simulink model "lab4p2b"  (R2023b)
settings: Solver=ode23tb  StartTime=0.0  StopTime=Tmdl  FixedStep=To/100  MaxStep=To/100  RelTol=1e-3
undefined symbols (not defined in the file or in its folder): an, dsc, T, To
settings Model: Creator=deniskirbaba  LastModifiedBy=Max

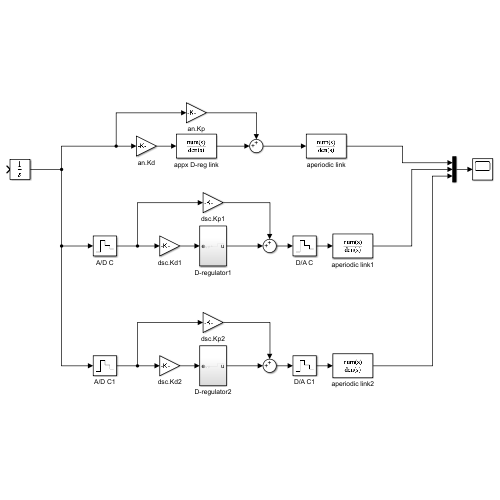
[thumbnail: Simulink's stored preview of the top-level diagram]
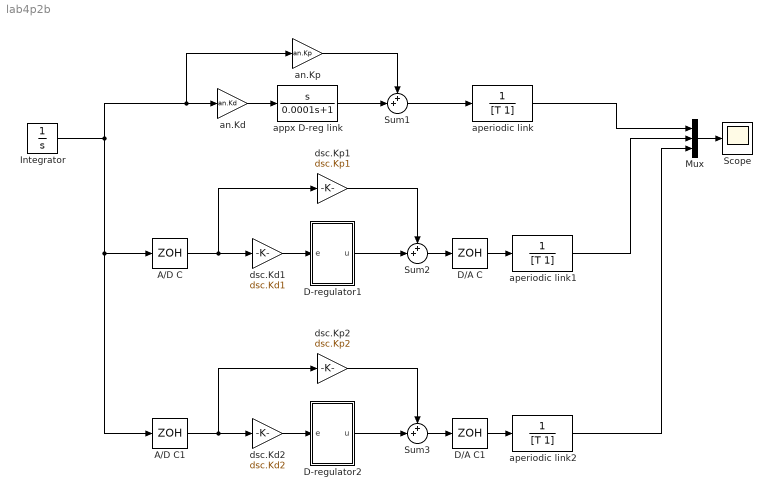
== system lab4p2b ==
  A/D C : ZeroOrderHold  SampleTime=To
  A/D C1 : ZeroOrderHold  SampleTime=To
  D-regulator1 : Subsystem
  D-regulator2 : Subsystem
  D/A C : ZeroOrderHold  SampleTime=To
  D/A C1 : ZeroOrderHold  SampleTime=To
  Integrator : Integrator  InitialCondition=1
  Mux : Mux  Inputs=3
  Scope : Scope
  Sum1 : Sum  Inputs=++|
  Sum2 : Sum  Inputs=++|
  Sum3 : Sum  Inputs=++|
  an.Kd : Gain  Gain=an.Kd
  an.Kp : Gain  Gain=an.Kp
  aperiodic link : TransferFcn  Denominator=[T 1]
  aperiodic link1 : TransferFcn  Denominator=[T 1]
  aperiodic link2 : TransferFcn  Denominator=[T 1]
  appx D-reg link : TransferFcn  Numerator=[1 0]  Denominator=[0.0001 1]
  dsc.Kd1 : Gain  Gain=dsc.Kd1
  dsc.Kd2 : Gain  Gain=dsc.Kd2
  dsc.Kp1 : Gain  Gain=dsc.Kp1
  dsc.Kp2 : Gain  Gain=dsc.Kp2
  wires:
  an.Kd/1 -> appx D-reg link/1
  Mux/1 -> Scope/1
  appx D-reg link/1 -> Sum1/2
  an.Kp/1 -> Sum1/1
  Sum1/1 -> aperiodic link/1
  aperiodic link/1 -> Mux/1
  dsc.Kd1/1 -> D-regulator1/1(e)
  D-regulator1/1(u) -> Sum2/2
  A/D C/1 -> dsc.Kp1/1, dsc.Kd1/1
  dsc.Kp1/1 -> Sum2/1
  Sum2/1 -> D/A C/1
  aperiodic link1/1 -> Mux/2
  D/A C/1 -> aperiodic link1/1
  aperiodic link2/1 -> Mux/3
  D/A C1/1 -> aperiodic link2/1
  dsc.Kp2/1 -> Sum3/1
  A/D C1/1 -> dsc.Kp2/1, dsc.Kd2/1
  Sum3/1 -> D/A C1/1
  dsc.Kd2/1 -> D-regulator2/1(e)
  D-regulator2/1(u) -> Sum3/2
  Integrator/1 -> A/D C1/1, A/D C/1, an.Kp/1, an.Kd/1

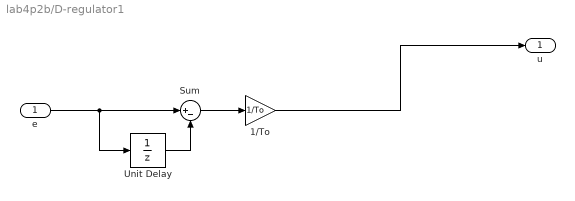
== system lab4p2b/D-regulator1 ==
  e : Inport
  1/To : Gain  Gain=1/To
  Sum : Sum  Inputs=|+-
  Unit Delay : UnitDelay  SampleTime=To  HasFrameUpgradeWarning=on
  u : Outport
  wires:
  1/To/1 -> u/1
  Unit Delay/1 -> Sum/2
  e/1 -> Unit Delay/1, Sum/1
  Sum/1 -> 1/To/1

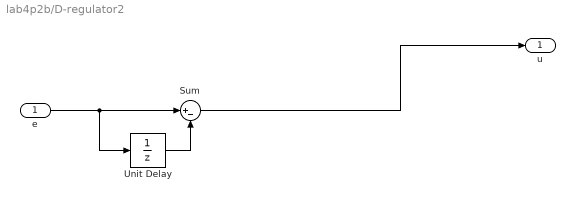
== system lab4p2b/D-regulator2 ==
  e : Inport
  Sum : Sum  Inputs=|+-
  Unit Delay : UnitDelay  SampleTime=To  HasFrameUpgradeWarning=on
  u : Outport
  wires:
  Sum/1 -> u/1
  Unit Delay/1 -> Sum/2
  e/1 -> Unit Delay/1, Sum/1
